simulink model "vdptop"  (Simulink 7.0)
settings: Solver=ode3  SolverMode=SingleTasking  StartTime=0.0  StopTime=20  RelTol=1e-3  AbsTol=1e-6
libraries: simulink x1
Description:
  | The van der Pol Equation
  | 
  | This is a simulation of a nonlinear second order system.
settings Model: Creator=The MathWorks Inc.  LastModifiedBy=colinlea  ExtModeAutoUpdateStatusClock=off
settings DataIOCC: ExternalInput=[]  InitialState=[]  LimitDataPoints=off  SaveOutput=off  SaveTime=off
settings OptimizationCC: BlockReduction=off  BooleanDataType=off  InlineParams=on  InlineInvariantSignals=on  BufferReusableBoundary=off
settings DebuggingCC: SaveWithParameterizedLinksMsg=none  SolverPrmCheckMsg=none  MultiTaskDSMMsg=warning  MultiTaskCondExecSysMsg=none  BusObjectLabelMismatch=none  StrictBusMsg=ErrorLevel1
settings HardwareCC: TargetUnknown=on
settings ModelReferenceCC: UpdateModelReferenceTargets=IfOutOfDate
settings RTWCC: IncludeERTFirstTime=on
settings GRTTargetCC: TargetFcnLib=ansi_tfl_tmw.mat

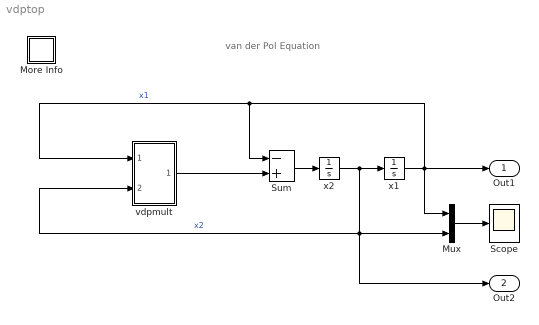
== system vdptop ==
  note: van der Pol Equation
  More Info : Subsystem
      mask Display: disp('?')
  Mux : Mux  Inputs=2
  Scope : Scope
      settings: TickLabels=on  TimeRange=20  YMin=-3  YMax=3  DataFormat=Array
  Sum : Sum  Inputs=-+  OutDataType=sfix(16)  OutScaling=2^0  SaturateOnIntegerOverflow=on  InputSameDT=on
  vdpmult : Subsystem  TreatAsAtomicUnit=on
  x1 : Integrator  InitialCondition=2
  x2 : Integrator
  Out1 : Outport  OutDataType=sfix(16)  OutScaling=2^0  InitialOutput=0
  Out2 : Outport  Port=2  OutDataType=sfix(16)  OutScaling=2^0  InitialOutput=0
  wires:
  Sum/1 -> x2/1
  x2/1 -> x1/1, Mux/2, vdpmult/2(In2), Out2/1  "x2"
  x1/1 -> Out1/1, Mux/1, Sum/1, vdpmult/1(In1)  "x1"
  Mux/1 -> Scope/1
  vdpmult/1(Out1) -> Sum/2

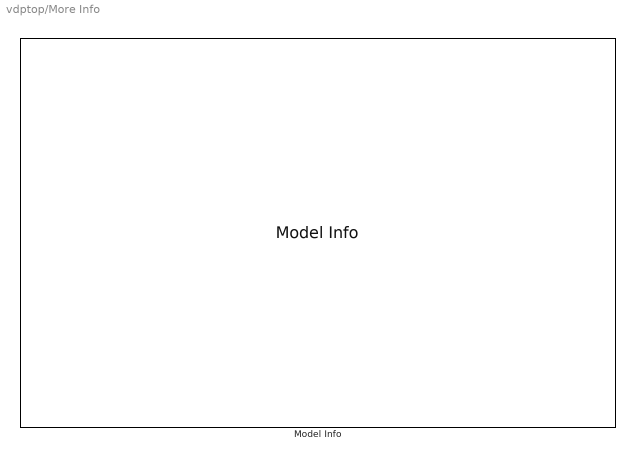
== system vdptop/More Info ==
  Model Info : simulink/Model-Wide Utilities/Model Info  InitialBlockCM=none  BlockCM=None  Frame=on  DisplayStringWithTags=|  HorizontalTextAlignment=Left  LeftAlignmentValue=0.02  SourceBlockDiagram=vdp  TagMaxNumber=20
      | Model Description:
      | -------------------
      | 
      | %<Description>

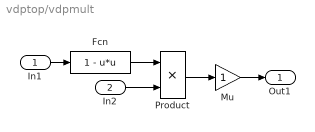
== system vdptop/vdpmult ==
  In1 : Inport
  In2 : Inport  Port=2
  Fcn : Fcn  Expr=1 - u*u
  Mu : Gain  ParameterDataType=sfix(16)  ParameterScaling=2^0  OutDataType=sfix(16)  OutScaling=2^0  SaturateOnIntegerOverflow=on
  Product : Product  OutDataType=sfix(16)  OutScaling=2^0  SaturateOnIntegerOverflow=on  RndMeth=Zero  InputSameDT=on
  Out1 : Outport
  wires:
  Product/1 -> Mu/1
  Fcn/1 -> Product/1
  In1/1 -> Fcn/1
  In2/1 -> Product/2
  Mu/1 -> Out1/1
